simulink model "HW2_es4"  (R2024a)
settings: Solver=VariableStepAuto  StartTime=0.0  StopTime=4  RelTol=1e-3
values from neighbouring files (symbols this model uses):
  Ts = 0.02    [H2_es4.m]
libraries: robotmobilelib x1
settings Model: Creator=Strix  LastModifiedBy=Strix

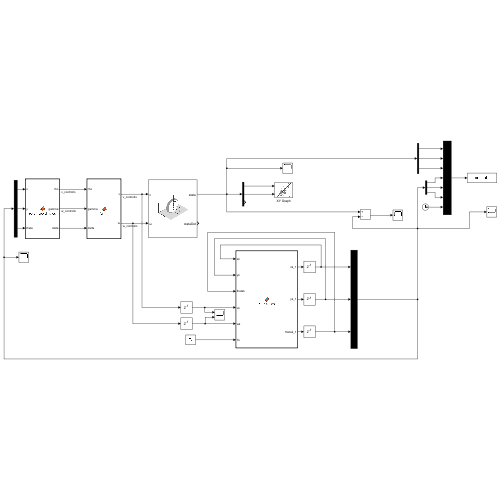
[thumbnail: Simulink's stored preview of the top-level diagram]
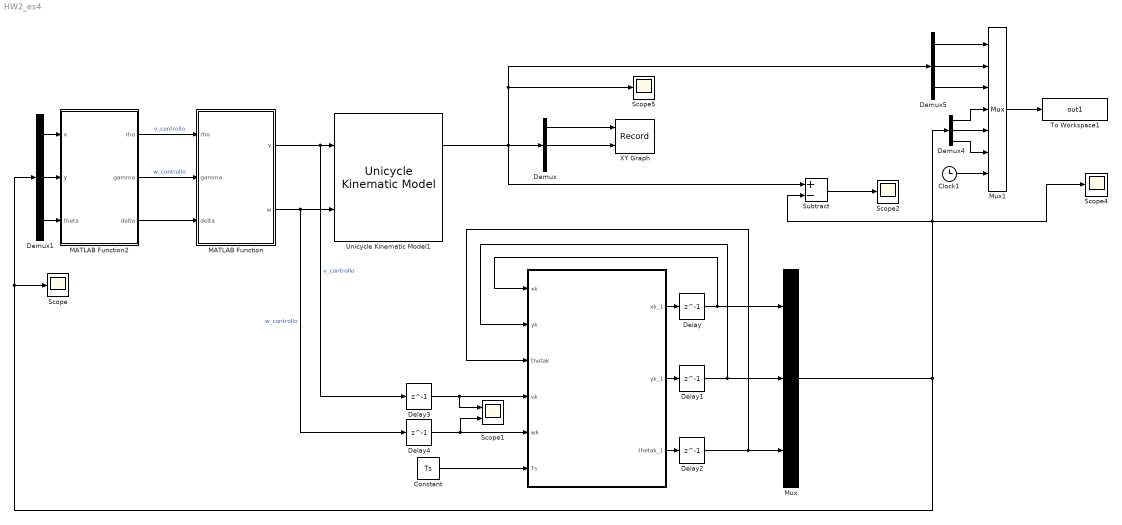
== system HW2_es4 ==
  " " : MATLAB Function  TreatAsAtomicUnit=on  SystemSampleTime=Ts
  Clock1 : Clock
  Constant : Constant  Value=Ts
  Delay : Delay  DelayLength=1  InitialCondition=2  InputProcessing=Columns as channels (frame based)
  Delay1 : Delay  DelayLength=1  InitialCondition=1  InputProcessing=Columns as channels (frame based)
  Delay2 : Delay  DelayLength=1  InitialCondition=pi/4  InputProcessing=Columns as channels (frame based)
  Delay3 : Delay  DelayLength=1  InitialCondition=2  InputProcessing=Columns as channels (frame based)
  Delay4 : Delay  DelayLength=1  InitialCondition=2  InputProcessing=Columns as channels (frame based)
  Demux{,1,4..5} (4 alike) : Demux  Outputs=3
  MATLAB Function : MATLAB Function  TreatAsAtomicUnit=on  SystemSampleTime=Ts
  MATLAB Function2 : MATLAB Function  TreatAsAtomicUnit=on  SystemSampleTime=Ts
  Mux : Mux  Inputs=3
  Mux1 : Mux  Inputs=7
  Scope{,2,4..5} (4 alike) : Scope
  Scope1 : Scope  NumInputPorts=2
  Subtract : Sum  Inputs=+-
  To Workspace1 : ToWorkspace  VariableName=out1  SampleTime=-1
  Unicycle Kinematic Model1 : robotmobilelib/Unicycle Kinematic Model  VehicleInputs=Vehicle Speed & Heading Angular Velocity  WheelRadius=0.1  WheelSpeedRange=[-Inf Inf]  InitialState=qi  SimulateUsing=Interpreted execution
  XY Graph : Record  FileSettingsInternal="{\"entries\":[{\"content\":{\"excelSettings\":{\"content\":{},\"type\":\"Streamout.ExcelSettings\"}},\"type\":\"Streamout.FileSettingStorage\",\"uuid\":\"\"}],\"packageUris\":[\"http:\\/\\/schema.mathworks.com\\/mf0\\/streamout_blocks\\/R2020a\"],\"version\":\"1.0\"}"  Layout=[1 1]  SignalsInternal="{\"entries\":[{\"content\":{\"signals\":[{\"content\":{\"blockPath\":[],\"dimensions\":[1],\"domain\":\"\",\"lineColor\":\"#a2142f\",\"plots\":[ 1 ],\"port\":1,\"sid\":[\"\"],\"signalID\":1,\"signalName\":\"Demux:1\"},\"type\":\"RecordBlkView.Signal\",\"uuid\":\"\"},{\"content\":{\"blockPath\":[],\"dimensions\":[1],\"domain\":\"\",\"lineColor\":\"#139fff\",\"plots\":[ 1 ],\"port\":2,\"sid\":[\"\"],\"signalID\":2,\"signalName\":\"Demux:2\"},\"type\":\"RecordBlkView.Signal\",\"uuid\":\"\"}]},\"type\":\"RecordBlkView.InputSignals\",\"uuid\":\"\"}],\"packageUris\":[\"http:\\/\\/schema.mathworks.com\\/mf0\\/streamout_blocks\\/R2020a\"],\"version\":\"1.0\"}"  VisualizationBindings="{\"xyplotplugin\":{\"info\":[{\"series\":[{\"bindingParametersList\":[{\"parameter\":\"X-Axis\",\"signalID\":1,\"signalName\":\"Demux:1\"},{\"parameter\":\"Y-Axis\",\"signalID\":2,\"signalName\":\"Demux:2\"}],\"seriesID\":0}],\"subplotID\":1}]}}"  CompatibilityTag=XY
  wires:
  Mux1/1 -> To Workspace1/1
  MATLAB Function/2(w) -> Delay4/1, Unicycle Kinematic Model1/2  "w_controllo"
  Demux/2 -> XY Graph/2
  Demux/1 -> XY Graph/1
  Demux5/1 -> Mux1/1
  Demux5/2 -> Mux1/2
  Demux5/3 -> Mux1/3
  Clock1/1 -> Mux1/7
  MATLAB Function2/1(rho) -> MATLAB Function/1(rho)  "v_controllo"
  MATLAB Function2/2(gamma) -> MATLAB Function/2(gamma)  "w_controllo"
  MATLAB Function2/3(delta) -> MATLAB Function/3(delta)
  Demux1/2 -> MATLAB Function2/2(y)
  Demux1/3 -> MATLAB Function2/3(theta)
  Demux1/1 -> MATLAB Function2/1(x)
  Constant/1 -> " "/6(Ts)
  " "/2(yk_1) -> Delay1/1
  " "/1(xk_1) -> Delay/1
  " "/3(thetak_1) -> Delay2/1
  Demux4/2 -> Mux1/5
  Demux4/1 -> Mux1/4
  Demux4/3 -> Mux1/6
  Unicycle Kinematic Model1/1 -> Scope5/1, Demux5/1, Subtract/1, Demux/1
  MATLAB Function/1(v) -> Delay3/1, Unicycle Kinematic Model1/1  "v_controllo"
  Subtract/1 -> Scope2/1
  Delay1/1 -> " "/2(yk), Mux/2
  Delay/1 -> " "/1(xk), Mux/1
  Mux/1 -> Demux1/1, Scope/1, Scope4/1, Subtract/2, Demux4/1
  Delay2/1 -> " "/3(thetak), Mux/3
  Delay3/1 -> " "/4(vk), Scope1/1
  Delay4/1 -> Scope1/2, " "/5(wk)

== matlab function HW2_es4/MATLAB Function ==
  data: rho input; v output; gamma input; w output; delta input
function [v,w] = fcn_1(rho,gamma,delta)
k1=3;
k2=3;
k3=1;

v=k1*rho*cos(gamma)*(1+k3*delta/gamma);

w=k2*gamma+k1*rho*sin(gamma);

== matlab function HW2_es4/MATLAB Function2 ==
  data: x input; rho output; y input; gamma output; theta input; delta output
function [rho,gamma,delta] = polar_coordinates(x,y,theta)

rho=sqrt(x^2+y^2);
gamma=atan2(y,x)-theta;
delta=gamma+theta;

end

== matlab function HW2_es4/  ==
  data: xk input; yk input; thetak input; xk_1 output; yk_1 output; thetak_1 output; vk input; wk input; Ts input
function [xk_1,yk_1,thetak_1] = RungeKutta(xk, yk, thetak, vk, wk, Ts)

xk_1=xk+vk*Ts*cos(thetak+wk*Ts/2);
yk_1=yk+vk*Ts*sin(thetak+wk*Ts/2);
thetak_1=thetak+wk*Ts;

end
